simulink model "model_step"  (R2024b)
settings: Solver=VariableStepAuto  StartTime=0.0  StopTime=10.0  RelTol=1e-3
values from neighbouring files (symbols this model uses):
  denC = denCA    [carson.m]
  denG = G.Denominator{1}    [carson.m]
  numC = numCA    [carson.m]
  numG = G.Numerator{1}    [carson.m]
settings Model: Creator=carso  LastModifiedBy=carso

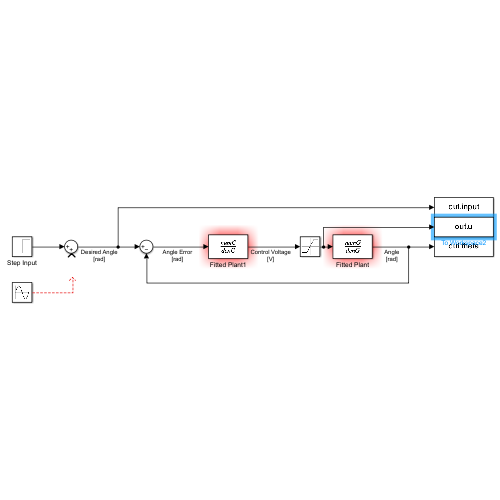
[thumbnail: Simulink's stored preview of the top-level diagram]
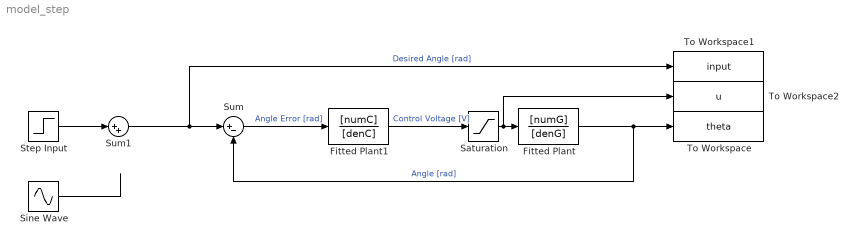
== system model_step ==
  Fitted Plant : TransferFcn  Numerator=[numG]  Denominator=[denG]
  Fitted Plant1 : TransferFcn  Numerator=[numC]  Denominator=[denC]
  Saturation : Saturate  UpperLimit=15  LowerLimit=-15
  Sine Wave : Sin  Frequency=0.73  SampleTime=0
  Step Input : Step  After=0.5  SampleTime=0
  Sum : Sum  Inputs=|+-
  Sum1 : Sum  Inputs=|++
  To Workspace : ToWorkspace  VariableName=theta  SaveFormat=Timeseries  SampleTime=-1
  To Workspace1 : ToWorkspace  VariableName=input  SaveFormat=Timeseries  SampleTime=-1
  To Workspace2 : ToWorkspace  VariableName=u  SaveFormat=Timeseries  SampleTime=-1
  wires:
  Fitted Plant1/1 -> Saturation/1  "Control Voltage [V]"
  Sum/1 -> Fitted Plant1/1  "Angle Error [rad]"
  Fitted Plant/1 -> Sum/2, To Workspace/1  "Angle [rad]"
  Step Input/1 -> Sum1/1
  Sine Wave/1 -> ?
  Sum1/1 -> To Workspace1/1, Sum/1  "Desired Angle [rad]"
  Saturation/1 -> To Workspace2/1, Fitted Plant/1
